simulink subsystem "Lift_Cruise_Reference_Inputs"  (R2024b)
settings: Solver=VariableStepAuto  StartTime=0.0  StopTime=10.0  RelTol=1e-3
undefined symbols (not defined in the file or in its folder): SimPar
libraries: DoubletsLib x3, starslibMathOperations x1
settings Model: Creator=tbritton  LastModifiedBy=adcl
settings SolverCC: AlgebraicLoopSolver=TrustRegion
settings OptimizationCC: ReuseModelBlockBuffer=off
settings DebuggingCC: UnconnectedInputMsg=warning  UnconnectedOutputMsg=warning  UnconnectedLineMsg=warning
settings ModelReferenceCC: EnableRefExpFcnMdlSchedulingChecks=on
settings RTWCC: GPUComputeCapability=3.5  DLArmComputeVersion=19.05

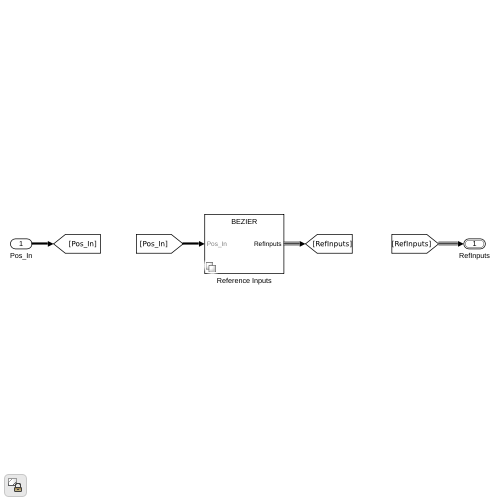
[thumbnail: Simulink's stored preview of the top-level diagram]
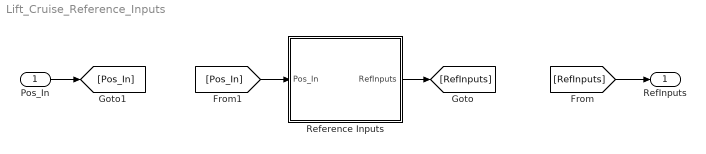
== system Lift_Cruise_Reference_Inputs ==
  Pos_In : Inport
  Reference Inputs : Subsystem  Variant=on
  RefInputs : Outport  OutDataTypeStr=Bus: BUS_REF_INPUT  VectorParamsAs1DForOutWhenUnconnected=off
  wires:
  [RefInputs] -> RefInputs/1
  Reference Inputs/1(RefInputs) -> [RefInputs]
  [Pos_In] -> Reference Inputs/1(Pos_In)
  Pos_In/1 -> [Pos_In]

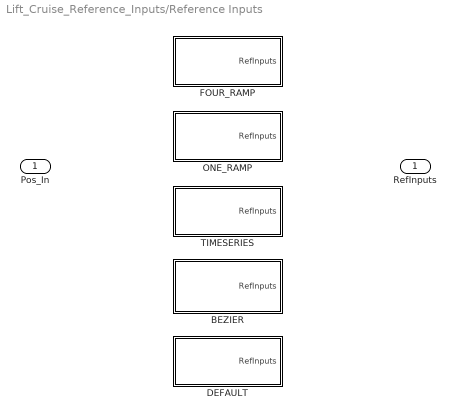
== system Lift_Cruise_Reference_Inputs/Reference Inputs ==
  Pos_In : Inport
  BEZIER : Subsystem  VariantControl=GVS_REFINPUT_TYPE_BEZIER
  DEFAULT : Subsystem  VariantControl=GVS_REFINPUT_TYPE_DEFAULT
  FOUR_RAMP : Subsystem  VariantControl=GVS_REFINPUT_TYPE_4RAMP
  ONE_RAMP : Subsystem  VariantControl=GVS_REFINPUT_TYPE_1RAMP
  TIMESERIES : Subsystem  VariantControl=GVS_REFINPUT_TYPE_TIMESERIES
  RefInputs : Outport  OutDataTypeStr=Bus: BUS_REF_INPUT  VectorParamsAs1DForOutWhenUnconnected=off

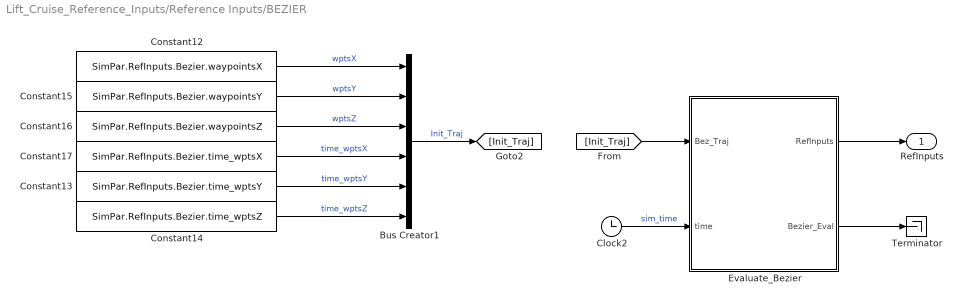
== system Lift_Cruise_Reference_Inputs/Reference Inputs/BEZIER ==
  Bus Creator1 : BusCreator  Inputs=6
  Clock2 : Clock
  Constant12 : Constant  Value=SimPar.RefInputs.Bezier.waypointsX  SampleTime=-1
  Constant13 : Constant  Value=SimPar.RefInputs.Bezier.time_wptsY  VectorParams1D=off  SampleTime=-1
  Constant14 : Constant  Value=SimPar.RefInputs.Bezier.time_wptsZ  VectorParams1D=off  SampleTime=-1
  Constant15 : Constant  Value=SimPar.RefInputs.Bezier.waypointsY  SampleTime=-1
  Constant16 : Constant  Value=SimPar.RefInputs.Bezier.waypointsZ  SampleTime=-1
  Constant17 : Constant  Value=SimPar.RefInputs.Bezier.time_wptsX  VectorParams1D=off  SampleTime=-1
  Evaluate_Bezier : Subsystem  mask{tlen_max=1}
      mask prompts: tlen_max "Enter the length of time vector:"
  Terminator : Terminator
  RefInputs : Outport
  wires:
  Evaluate_Bezier/2(Bezier_Eval) -> Terminator/1
  Evaluate_Bezier/1(RefInputs) -> RefInputs/1
  [Init_Traj] -> Evaluate_Bezier/1(Bez_Traj)
  Bus Creator1/1 -> [Init_Traj]  "Init_Traj"
  Clock2/1 -> Evaluate_Bezier/2(time)  "sim_time"
  Constant14/1 -> Bus Creator1/6  "time_wptsZ"
  Constant13/1 -> Bus Creator1/5  "time_wptsY"
  Constant17/1 -> Bus Creator1/4  "time_wptsX"
  Constant15/1 -> Bus Creator1/2  "wptsY"
  Constant12/1 -> Bus Creator1/1  "wptsX"
  Constant16/1 -> Bus Creator1/3  "wptsZ"

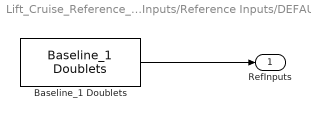
== system Lift_Cruise_Reference_Inputs/Reference Inputs/DEFAULT ==
  Baseline_1 Doublets : DoubletsLib/Baseline_1 Doublets  SystemSampleTime=-1  VariantActivationTime=update diagram  AllowFlexibleInterface=on  Latency=0  AutoFrameSizeCalculation=off
  RefInputs : Outport
  wires:
  Baseline_1 Doublets/1 -> RefInputs/1

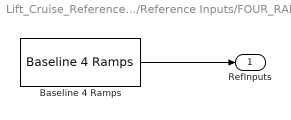
== system Lift_Cruise_Reference_Inputs/Reference Inputs/FOUR_RAMP ==
  Baseline 4 Ramps : DoubletsLib/Baseline 4 Ramps  SystemSampleTime=-1  VariantActivationTime=update diagram  Latency=0  AutoFrameSizeCalculation=off
  RefInputs : Outport
  wires:
  Baseline 4 Ramps/1 -> RefInputs/1

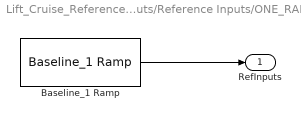
== system Lift_Cruise_Reference_Inputs/Reference Inputs/ONE_RAMP ==
  Baseline_1 Ramp : DoubletsLib/Baseline_1 Ramp  SystemSampleTime=-1  VariantActivationTime=update diagram  Latency=0  AutoFrameSizeCalculation=off
  RefInputs : Outport
  wires:
  Baseline_1 Ramp/1 -> RefInputs/1

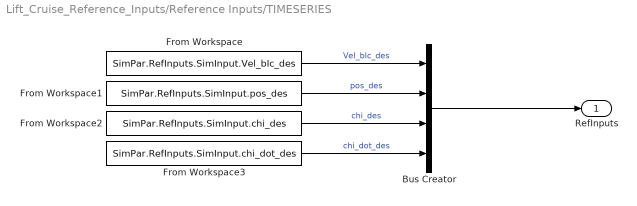
== system Lift_Cruise_Reference_Inputs/Reference Inputs/TIMESERIES ==
  Bus Creator : BusCreator  Inputs=4
  From Workspace : FromWorkspace  VariableName=SimPar.RefInputs.SimInput.Vel_bIc_des  OutputAfterFinalValue=Holding final value
  From Workspace1 : FromWorkspace  VariableName=SimPar.RefInputs.SimInput.pos_des  OutputAfterFinalValue=Holding final value
  From Workspace2 : FromWorkspace  VariableName=SimPar.RefInputs.SimInput.chi_des  OutputAfterFinalValue=Holding final value
  From Workspace3 : FromWorkspace  VariableName=SimPar.RefInputs.SimInput.chi_dot_des  OutputAfterFinalValue=Holding final value
  RefInputs : Outport
  wires:
  Bus Creator/1 -> RefInputs/1
  From Workspace3/1 -> Bus Creator/4  "chi_dot_des"
  From Workspace2/1 -> Bus Creator/3  "chi_des"
  From Workspace1/1 -> Bus Creator/2  "pos_des"
  From Workspace/1 -> Bus Creator/1  "Vel_bIc_des"

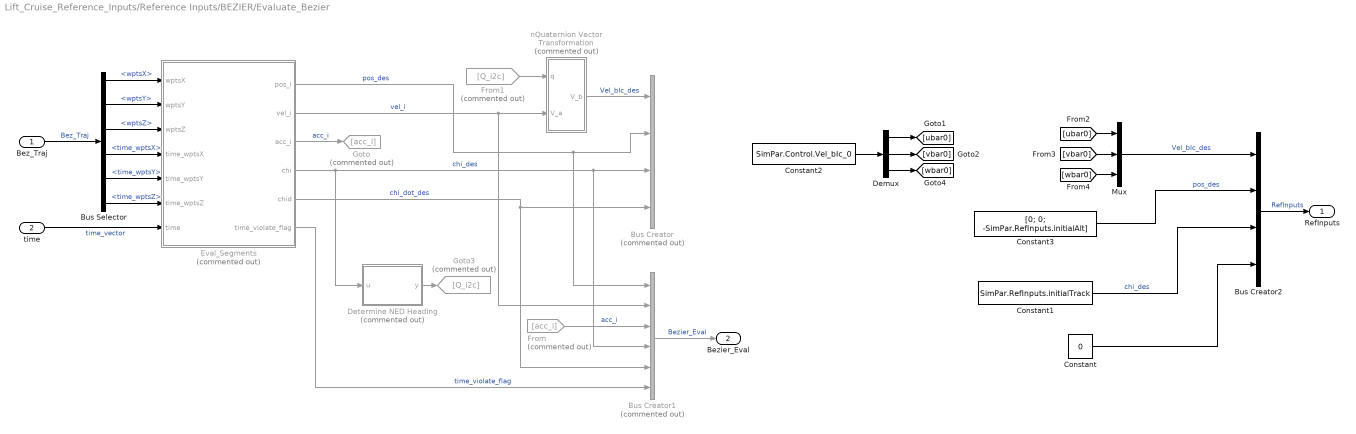
== system Lift_Cruise_Reference_Inputs/Reference Inputs/BEZIER/Evaluate_Bezier ==
  Bez_Traj : Inport
  time : Inport  Port=2
  Bus Creator : BusCreator  Commented=on  Inputs=4
  Bus Creator1 : BusCreator  Commented=on  Inputs=6
  Bus Creator2 : BusCreator  Inputs=4
  Bus Selector : BusSelector  OutputSignals=wptsX,wptsY,wptsZ,time_wptsX,time_wptsY,time_wptsZ
  Constant : Constant  Value=0
  Constant1 : Constant  Value=SimPar.RefInputs.initialTrack
  Constant2 : Constant  Value=SimPar.Control.Vel_bIc_0
  Constant3 : Constant  Value=[0; 0; -SimPar.RefInputs.initialAlt]
  Demux : Demux  Outputs=3
  Determine NED Heading : MATLAB Function  Commented=on  TreatAsAtomicUnit=on
  Eval_Segments : MATLAB Function  Commented=on  TreatAsAtomicUnit=on
  From : From  Commented=on  GotoTag=acc_i
  From1 : From  Commented=on  GotoTag=Q_i2c
  Goto : Goto  Commented=on  GotoTag=acc_i
  Goto3 : Goto  Commented=on  GotoTag=Q_i2c
  Mux : Mux  Inputs=3
  nQuaternion Vector Transformation : Subsystem  Commented=on
  RefInputs : Outport
  Bezier_Eval : Outport  Port=2
  wires:
  Constant/1 -> Bus Creator2/4
  Demux/2 -> [vbar0]
  Constant2/1 -> Demux/1
  Demux/1 -> [ubar0]
  Demux/3 -> [wbar0]
  [wbar0] -> Mux/3
  [ubar0] -> Mux/1
  [vbar0] -> Mux/2
  Mux/1 -> Bus Creator2/1  "Vel_bIc_des"
  Constant1/1 -> Bus Creator2/3  "chi_des"
  Constant3/1 -> Bus Creator2/2  "pos_des"
  Eval_Segments/6(time_violate_flag) -> Bus Creator1/6  "time_violate_flag"
  From/1 -> Bus Creator1/3  "acc_i"
  Eval_Segments/3(acc_i) -> Goto/1  "acc_i"
  Bus Creator1/1 -> Bezier_Eval/1  "Bezier_Eval"
  Bus Creator2/1 -> RefInputs/1  "RefInputs"
  Bus Selector/4 -> Eval_Segments/4(time_wptsX)  "<time_wptsX>"
  From1/1 -> nQuaternion Vector Transformation/1(q)
  Determine NED Heading/1(y) -> Goto3/1
  Eval_Segments/2(vel_i) -> Bus Creator1/2, nQuaternion Vector Transformation/2(V_a)  "vel_i"
  Bez_Traj/1 -> Bus Selector/1  "Bez_Traj"
  Bus Selector/2 -> Eval_Segments/2(wptsY)  "<wptsY>"
  Bus Selector/3 -> Eval_Segments/3(wptsZ)  "<wptsZ>"
  time/1 -> Eval_Segments/7(time)  "time_vector"
  Bus Selector/1 -> Eval_Segments/1(wptsX)  "<wptsX>"
  Eval_Segments/4(chi) -> Bus Creator/3, Bus Creator1/4, Determine NED Heading/1(u)  "chi_des"
  Eval_Segments/5(chid) -> Bus Creator/4, Bus Creator1/5  "chi_dot_des"
  Bus Selector/5 -> Eval_Segments/5(time_wptsY)  "<time_wptsY>"
  Eval_Segments/1(pos_i) -> Bus Creator1/1, Bus Creator/2  "pos_des"
  Bus Selector/6 -> Eval_Segments/6(time_wptsZ)  "<time_wptsZ>"
  nQuaternion Vector Transformation/1(V_b) -> Bus Creator/1  "Vel_bIc_des"

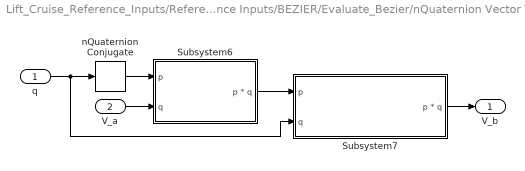
== system Lift_Cruise_Reference_Inputs/Reference Inputs/BEZIER/Evaluate_Bezier/nQuaternion Vector Transformation ==
  q : Inport  PortDimensions=[4,tlen_max]
  V_a : Inport  Port=2  PortDimensions=[3,tlen_max]
  Subsystem6 : Subsystem  mask(Quat Mult for two special sets of quaternions){nQuat=tlen_max}
      mask prompts: nQuat "Number of quaternions in input"
      mask help:
      | Quaternion multiplication of two sets of quaternions
      | inputted by 2 (4 x nQuat) matrices. First element assumed
      | zero of second Quaternion.  Input only last three elements
      | of second quaternion.  Used in Qtrans' first quaternion
      | multiplication
      mask Display:
      | disp('n-Quat Mult\n q0=0')
      | port_label('input',1,'p')
      | port_label('input',2,'q')
      | port_label('output',1,'p*q')
  Subsystem7 : Subsystem  mask(Quat Mult for two sets of quaternions){nQuat=tlen_max}
      mask prompts: nQuat "Number of quaternions in input"
      mask help:
      | Quaternion multiplication of two sets of quaternions
      | inputted by 2 (4 x nQuat) matrices.  Outputs only last
      | three elements of product.  Used in QTrans' second
      | multiplication
      mask Display:
      | disp('n-Quat Mult\n 1st Row\nRemoved')
      | port_label('input',1,'p')
      | port_label('input',2,'q')
      | port_label('output',1,'p*q')
  nQuaternion Conjugate : starslibMathOperations/nQuaternion Conjugate  n=tlen_max
  V_b : Outport  PortDimensions=[3,tlen_max]
  wires:
  V_a/1 -> Subsystem6/2(q)
  Subsystem7/1(p * q) -> V_b/1
  Subsystem6/1(p * q) -> Subsystem7/1(p)
  nQuaternion Conjugate/1 -> Subsystem6/1(p)
  q/1 -> Subsystem7/2(q), nQuaternion Conjugate/1

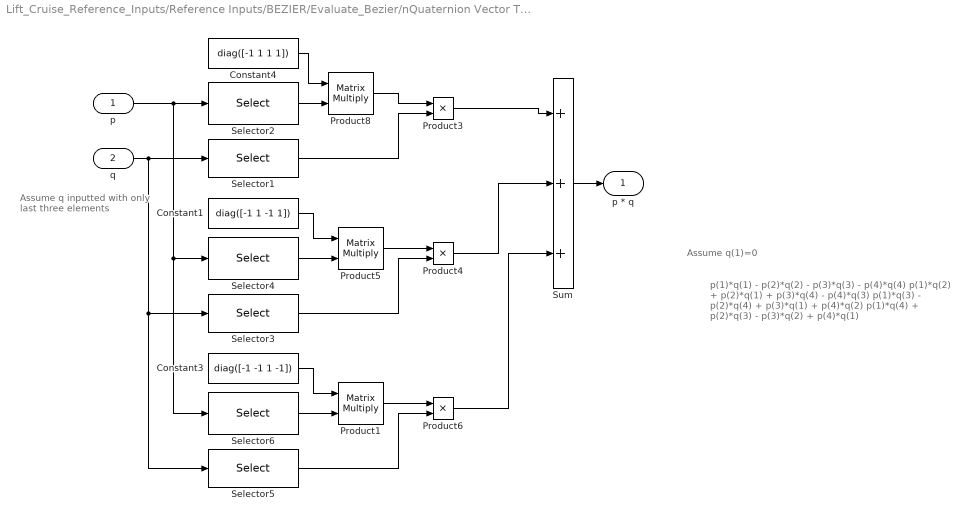
== system Lift_Cruise_Reference_Inputs/Reference Inputs/BEZIER/Evaluate_Bezier/nQuaternion Vector Transformation/Subsystem6 ==
  note: p(1)*q(1) - p(2)*q(2) - p(3)*q(3) - p(4)*q(4)
      |
      | p(1)*q(2) + p(2)*q(1) + p(3)*q(4) - p(4)*q(3)
      |
      | p(1)*q(3) - p(2)*q(4) + p(3)*q(1) + p(4)*q(2)
      |
      | p(1)*q(4) + p(2)*q(3) - p(3)*q(2) + p(4)*q(1)
  note: Assume q(1)=0
  note: Assume q
      | inputted with only
      | last three elements
  p : Inport  PortDimensions=[4,nQuat]
  q : Inport  Port=2  PortDimensions=[3,nQuat]
  Constant1 : Constant  Value=diag([-1 1 -1 1])  VectorParams1D=off
  Constant3 : Constant  Value=diag([-1 -1 1 -1])  VectorParams1D=off
  Constant4 : Constant  Value=diag([-1 1 1 1])  VectorParams1D=off
  Product1 : Product  Multiplication=Matrix(*)  RndMeth=Zero
  Product3 : Product  RndMeth=Zero
  Product4 : Product  RndMeth=Zero
  Product5 : Product  Multiplication=Matrix(*)  RndMeth=Zero
  Product6 : Product  RndMeth=Zero
  Product8 : Product  Multiplication=Matrix(*)  RndMeth=Zero
  Selector1 : Selector  NumberOfDimensions=2  InputPortWidth=3  IndexOptions=Index vector (dialog),Select all  Indices=[1 1 2 3],1  OutputSizes=1,1
  Selector2 : Selector  NumberOfDimensions=2  InputPortWidth=3  IndexOptions=Index vector (dialog),Select all  Indices=[2 1 1 1],1  OutputSizes=1,1
  Selector3 : Selector  NumberOfDimensions=2  InputPortWidth=3  IndexOptions=Index vector (dialog),Select all  Indices=[2 3 3 2],1  OutputSizes=1,1
  Selector4 : Selector  NumberOfDimensions=2  InputPortWidth=3  IndexOptions=Index vector (dialog),Select all  Indices=[3 3 2 2],1  OutputSizes=1,1
  Selector5 : Selector  NumberOfDimensions=2  InputPortWidth=3  IndexOptions=Index vector (dialog),Select all  Indices=[3 2 1 1],1  OutputSizes=1,1
  Selector6 : Selector  NumberOfDimensions=2  InputPortWidth=3  IndexOptions=Index vector (dialog),Select all  Indices=[4 4 4 3],1  OutputSizes=1,1
  Sum : Sum  Inputs=+++
  p * q : Outport  PortDimensions=[4,nQuat]
  wires:
  Selector4/1 -> Product5/2
  Constant1/1 -> Product5/1
  Selector6/1 -> Product1/2
  Constant3/1 -> Product1/1
  Selector1/1 -> Product3/2
  Product5/1 -> Product4/1
  Selector3/1 -> Product4/2
  Product1/1 -> Product6/1
  Selector5/1 -> Product6/2
  Product3/1 -> Sum/1
  Product4/1 -> Sum/2
  Product6/1 -> Sum/3
  p/1 -> Selector2/1, Selector4/1, Selector6/1
  q/1 -> Selector1/1, Selector3/1, Selector5/1
  Sum/1 -> p * q/1
  Selector2/1 -> Product8/2
  Product8/1 -> Product3/1
  Constant4/1 -> Product8/1

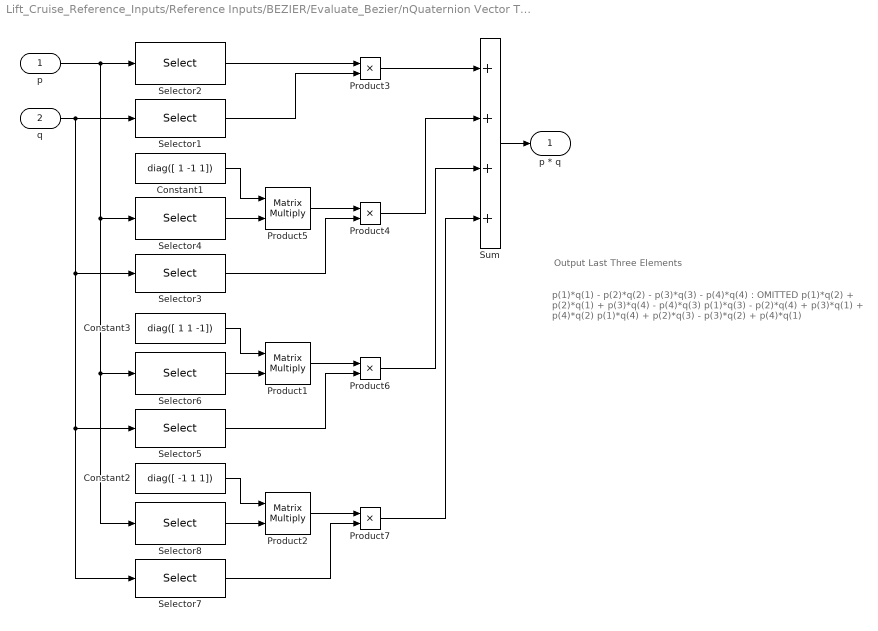
== system Lift_Cruise_Reference_Inputs/Reference Inputs/BEZIER/Evaluate_Bezier/nQuaternion Vector Transformation/Subsystem7 ==
  note: p(1)*q(1) - p(2)*q(2) - p(3)*q(3) - p(4)*q(4) :  OMITTED
      |
      | p(1)*q(2) + p(2)*q(1) + p(3)*q(4) - p(4)*q(3)
      |
      | p(1)*q(3) - p(2)*q(4) + p(3)*q(1) + p(4)*q(2)
      |
      | p(1)*q(4) + p(2)*q(3) - p(3)*q(2) + p(4)*q(1)
  note: Output Last Three Elements
  p : Inport  PortDimensions=[4,nQuat]
  q : Inport  Port=2  PortDimensions=[4,nQuat]
  Constant1 : Constant  Value=diag([ 1 -1 1])  VectorParams1D=off
  Constant2 : Constant  Value=diag([ -1 1 1])  VectorParams1D=off
  Constant3 : Constant  Value=diag([ 1 1 -1])  VectorParams1D=off
  Product1 : Product  Multiplication=Matrix(*)  RndMeth=Zero
  Product2 : Product  Multiplication=Matrix(*)  RndMeth=Zero
  Product{3..4,6..7} (4 alike) : Product  RndMeth=Zero
  Product5 : Product  Multiplication=Matrix(*)  RndMeth=Zero
  Selector1 : Selector  NumberOfDimensions=2  InputPortWidth=3  IndexOptions=Index vector (dialog),Select all  Indices=[ 2 3 4],1  OutputSizes=1,1
  Selector2 : Selector  NumberOfDimensions=2  InputPortWidth=3  IndexOptions=Index vector (dialog),Select all  Indices=[ 1 1 1],1  OutputSizes=1,1
  Selector3 : Selector  NumberOfDimensions=2  InputPortWidth=3  IndexOptions=Index vector (dialog),Select all  Indices=[ 1 4 3],1  OutputSizes=1,1
  Selector4 : Selector  NumberOfDimensions=2  InputPortWidth=3  IndexOptions=Index vector (dialog),Select all  Indices=[ 2 2 2],1  OutputSizes=1,1
  Selector5 : Selector  NumberOfDimensions=2  InputPortWidth=3  IndexOptions=Index vector (dialog),Select all  Indices=[ 4 1 2],1  OutputSizes=1,1
  Selector6 : Selector  NumberOfDimensions=2  InputPortWidth=3  IndexOptions=Index vector (dialog),Select all  Indices=[ 3 3 3],1  OutputSizes=1,1
  Selector7 : Selector  NumberOfDimensions=2  InputPortWidth=3  IndexOptions=Index vector (dialog),Select all  Indices=[ 3 2 1],1  OutputSizes=1,1
  Selector8 : Selector  NumberOfDimensions=2  InputPortWidth=3  IndexOptions=Index vector (dialog),Select all  Indices=[4 4 4],1  OutputSizes=1,1
  Sum : Sum  Inputs=++++
  p * q : Outport  PortDimensions=[3,nQuat]
  wires:
  Selector4/1 -> Product5/2
  Constant1/1 -> Product5/1
  Selector6/1 -> Product1/2
  Constant3/1 -> Product1/1
  Selector8/1 -> Product2/2
  Constant2/1 -> Product2/1
  Selector2/1 -> Product3/1
  Selector1/1 -> Product3/2
  Product5/1 -> Product4/1
  Selector3/1 -> Product4/2
  Product1/1 -> Product6/1
  Selector5/1 -> Product6/2
  Product2/1 -> Product7/1
  Selector7/1 -> Product7/2
  Product3/1 -> Sum/1
  Product4/1 -> Sum/2
  Product6/1 -> Sum/3
  Product7/1 -> Sum/4
  p/1 -> Selector2/1, Selector4/1, Selector6/1, Selector8/1
  q/1 -> Selector1/1, Selector3/1, Selector5/1, Selector7/1
  Sum/1 -> p * q/1

== matlab function Lift_Cruise_Reference_Inputs/Reference Inputs/BEZIER/Evaluate_Bezier/Determine NED Heading ==
  data: u input; y output double size=[4, tlen_max]
function y = fcn(u)

s = cos(u/2);
v = sin(u/2);
y = [s, 0*v, 0*v, v]';

== matlab function Lift_Cruise_Reference_Inputs/Reference Inputs/BEZIER/Evaluate_Bezier/Eval_Segments ==
  settings: updateMethod=CONTINUOUS  sampleTime=SimIn.Rate.Bezier_Sample
  data: wptsX input; wptsY input; wptsZ input; time_wptsX input; time_wptsY input; time_wptsZ input; time input; pos_i output size=[3 tlen_max]; vel_i output size=[3 tlen_max]; acc_i output size=[3 tlen_max]; chi output size=tlen_max; chid output size=tlen_max; time_violate_flag output
function [pos_i, vel_i, acc_i, chi, chid, time_violate_flag] = evalSegments_Sim(wptsX, wptsY, wptsZ, time_wptsX, time_wptsY, time_wptsZ, time)
% function Script: evalSegments.m

% *************************************************************************
% Description: This script is used to interrogate one (or more) particular 
% segments of cells (wayponts and time_wpts) for position, velocity and
% accelerations.  This requires computation of control points and then
% using these to interrogate an individual point.
%
% In:
%   wptsX, wptsY, wptsZ:  An N x M array where N = # of segments(waypoints) 
%               and M = number of derivatives (e.g., pos vel accel)
%   time_wptsX (Y,Z): Row vector: doubles with time points for each segment
%               (if input is from constant block with "Treat vector as 1-D"
%               checked, then uncheck to preserve row vector input). NOTE:
%               only first and last times must be consistant across X,Y,Z
%   time:       column vector of times at which to interrogate the
%               bezier information
%
% Out:
%   pos_i:              Bezier curve evaluated for position at the input time
%   vel_i:              Bezier curve evaluated for velocity at the input time
%   accel_i:            Bezier curve evaluated for acceleration at the input time
%   chi:                Computed heading frame angle
%   chid:               Computed heading frame angle derivative
%   time_violate_flag:  Flag denotes one or more times outside time_wpts,
%                       -1 => time less than start time,
%                       1 => time greater than stop time
%
% Created:
%   9/9/2022
%   Michael Acheson
%   NASA Langley Research Center, D316
%   Email: michael.j.acheson@nasa.gov
%
% Mods:
%   DD Month YYYY - Name : Description
%   10/14/2022 MJA Modified script to be capable of handling input time as
%   a vector (not just a scalar.)  This enables its' use for other than just
%   trajectory lookup (e.g. at current sim time) such as for use with DDP.
%   Note, the time_wpts (X,Y & Z)vectors are assumed to have identical start 
%   and end times but may have differing number of wpts.  Any input time
%   vector element that asks for a time lookup earlier than the first
%   time_wpt (or after the last time) is adjusted to "hold" the corresponding
%   first/last wpt time.

% *************************************************************************

% Check time vector length against mask size
tlen = length(time); % Determine number of input times

% Hardcode wpt dimensions (x,y,z & num derivatives)
N_dim = 3; % X, Y & Z axes
N_der = 3; % position, velocity and acceleration derivatives

% Check if any time is before or after the minimum/maximum wpts time 
% NOTE: the initial and final wpt_timeX, wpt_timeY, and wpt_timeZ times 
% are assumed to be equivalent
time_violate_flag = 0; % Flag used to output evaluation time outside time_wpts

time_lt_min = time < time_wptsX(1);
if any(time_lt_min)
   time(time_lt_min) = ones(sum(time_lt_min),1)*time_wptsX(1); 
   time_violate_flag = -1; % Specify time violation below first time_wpts vector component
end

time_grt_max = time > time_wptsX(end);
if any(time_grt_max)
   time(time_grt_max)   = ones(sum(time_grt_max),1)*time_wptsX(end);
   time_violate_flag    = 1; % Specify time violation above last time_wpts vector component
end

% Initialize outputs 
pos_i   = zeros(3,tlen);
vel_i   = zeros(3,tlen);
acc_i   = zeros(3,tlen);

% Perform for each axis
time_wpts = zeros(1,max([length(time_wptsX), length(time_wptsY), length(time_wptsZ)]));
waypoints = zeros(max([size(wptsX,1), size(wptsY,1), size(wptsZ,1)]),max([size(wptsX,2), size(wptsY,2), size(wptsZ,2)]));
for n_dim = 1:N_dim
    switch n_dim
        case 1
            waypoints = wptsX;
            time_wpts = time_wptsX;
        case 2
            waypoints = wptsY;
            time_wpts = time_wptsY;
        case 3
            waypoints = wptsZ;
            time_wpts = time_wptsZ;
    end
    
    % Locate the time of interest
    [ind_seg] = discretize(time, time_wpts);
    uniq_ind_seg = unique(ind_seg,'stable'); % Determines number of unique indices (and retains sort order)
    num_uniq_ind = length(uniq_ind_seg);
    
    for loop = 1:num_uniq_ind % Cycle thru each unique bin (to compute control points and evaluate)
        wpts        = [waypoints(uniq_ind_seg(loop),1:N_der); waypoints(uniq_ind_seg(loop)+1,1:N_der)];
        tint        = time_wpts(uniq_ind_seg(loop): uniq_ind_seg(loop)+1);
        loop_ind    = (ind_seg == uniq_ind_seg(loop));
        % Compute the control points for current dimension
        ctl         = nan(N_der*2,N_der);
        ctl(:,1)    = interpHermBern(wpts,tint);
        for n_der = 1:N_der-1
            ctl_1 = diffBernControl(ctl(:,1),tint,n_der);
            ctl(:,n_der+1) = [ctl_1;nan(n_der,1)];
        end

        % Using the control points, evaluate the curve at the prescribed time
        Q1              = ctl(:,1);
        Q1              = Q1(~isnan(Q1));
        pos_i(n_dim, loop_ind) = evalBernPoly(Q1,time(loop_ind),tint);
        Q2              = ctl(:,2);
        Q2              = Q2(~isnan(Q2));
        vel_i(n_dim, loop_ind) = evalBernPoly(Q2,time(loop_ind),tint);
        Q3              = ctl(:,3);
        Q3              = Q3(~isnan(Q3));
        acc_i(n_dim, loop_ind) = evalBernPoly(Q3,time(loop_ind),tint);
    end

end % End of for n_dim = 1:N_dim

% Find heading frame angle and derivative
chi     = atan2(vel_i(2,:),vel_i(1,:))';
tempval = vel_i(1,:).^2 + vel_i(2,:).^2;
delfdelx = -vel_i(2,:)./tempval;
delfdely =  vel_i(1,:)./tempval;
chid = (delfdelx.*acc_i(1,:))' + (delfdely.*acc_i(2,:))';

% Check for any NaNs in chid, if they occur, set chid vector element to zero
chid_nan_ind = isnan(chid);
if any(chid_nan_ind)
    chid(chid_nan_ind) = zeros(sum(chid_nan_ind),1);
end
